simulink library "libMdl_GnssDataCorrector"  (R2019b)
settings: Solver=VariableStepAuto  StartTime=0.0  StopTime=10.0  RelTol=1e-3
undefined symbols (not defined in the file): gnss_lever_arm, sample_time
libraries: libMdl_transformVect x2, libMdl_crossProdMat x1
settings Model: Creator=Hanno  LastModifiedBy=Hanno

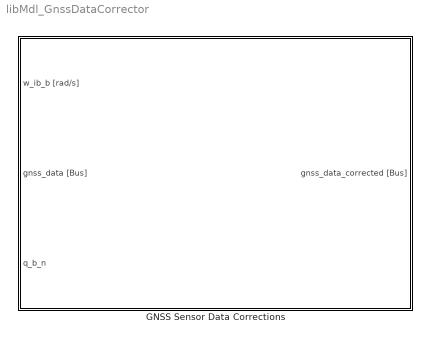
== system libMdl_GnssDataCorrector ==
  GNSS Sensor Data Corrections : Subsystem  mask(GNSS Sensor Data Corrections){mv_lever_arm=gnss_lever_arm, mv_sample_time=sample_time, mv_position_correction=on}
      mask prompts: mv_lever_arm "Lever Arm:"; mv_sample_time "Sample Time:"; mv_position_correction "Correct Position:"
      mask help: Lever Arm: Lever Arm Vector 'leverarm_s_b' in meters describing the mounting position of the sensor with respect to the body frame.
      mask Display:
      | if mv_position_correction
      |     pos_correction_str = 'on';
      | else
      |     pos_correction_str = 'off';
      | end % if
      | 
      | str1 = sprintf('\\color{black}{\\bfGNSS Data Correction}\n\n');
      | str2 = sprintf('Correct Position: %s\n',pos_correction_str);
      | str3 = sprintf('Sample Time: %0.3f',mv_sample_time);
      | 
      | str = [str1,str2,str3];
      | 
      | text( 0.5,0.5, ...
      |       str, ...
      |       'horizontalAlignment', 'center', ...
      |       'texmode','on' ...
      |     )

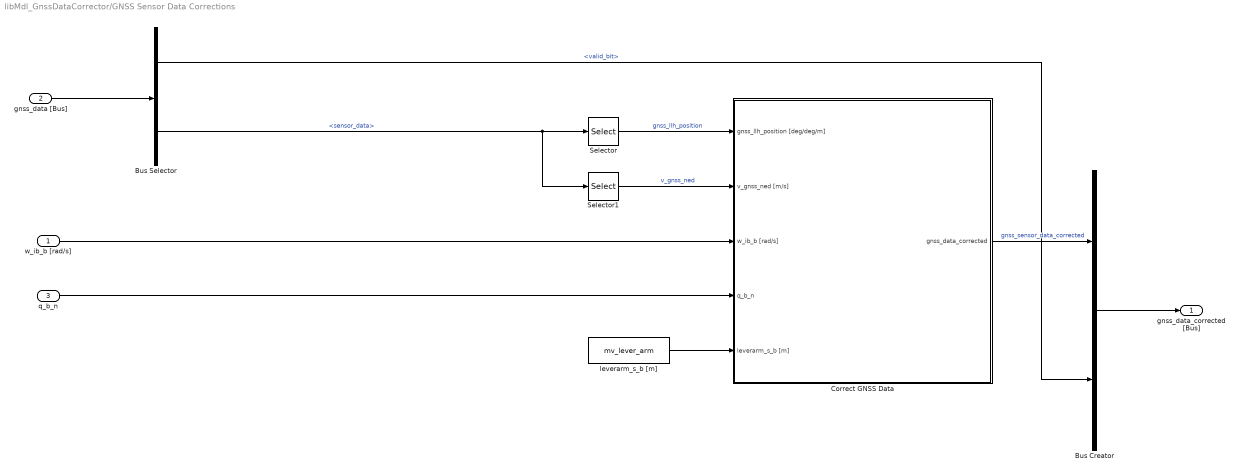
== system libMdl_GnssDataCorrector/GNSS Sensor Data Corrections ==
  w_ib_b [rad/s] : Inport
  gnss_data [Bus] : Inport  Port=2
  q_b_n : Inport  Port=3
  Bus Creator : BusCreator  Inputs=2
  Bus Selector : BusSelector  OutputSignals=valid_bit,sensor_data
  Correct GNSS Data : Subsystem  TreatAsAtomicUnit=on  SystemSampleTime=mv_sample_time
  Selector : Selector  InputPortWidth=7  IndexOptions=Index vector (dialog)  Indices=1:3  OutputSizes=1
  Selector1 : Selector  InputPortWidth=7  IndexOptions=Index vector (dialog)  Indices=4:6  OutputSizes=1
  leverarm_s_b [m] : Constant  Value=mv_lever_arm
  gnss_data_corrected [Bus] : Outport  VectorParamsAs1DForOutWhenUnconnected=off
  wires:
  gnss_data [Bus]/1 -> Bus Selector/1
  Bus Selector/2 -> Selector1/1, Selector/1  "<sensor_data>"
  Selector/1 -> Correct GNSS Data/1(gnss_llh_position [deg/deg/m])  "gnss_llh_position"
  Selector1/1 -> Correct GNSS Data/2(v_gnss_ned [m/s])  "v_gnss_ned"
  w_ib_b [rad/s]/1 -> Correct GNSS Data/3(w_ib_b [rad/s])
  q_b_n/1 -> Correct GNSS Data/4(q_b_n)
  leverarm_s_b [m]/1 -> Correct GNSS Data/5(leverarm_s_b [m])
  Bus Selector/1 -> Bus Creator/2  "<valid_bit>"
  Correct GNSS Data/1(gnss_data_corrected) -> Bus Creator/1  "gnss_sensor_data_corrected"
  Bus Creator/1 -> gnss_data_corrected [Bus]/1

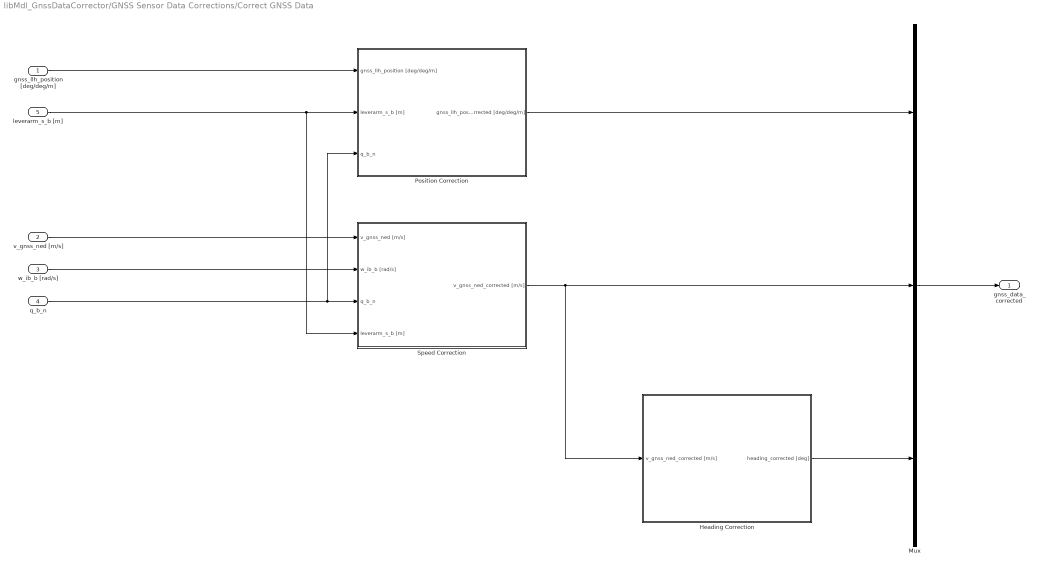
== system libMdl_GnssDataCorrector/GNSS Sensor Data Corrections/Correct GNSS Data ==
  gnss_llh_position [deg/deg/m] : Inport
  v_gnss_ned [m/s] : Inport  Port=2
  w_ib_b [rad/s] : Inport  Port=3
  q_b_n : Inport  Port=4
  leverarm_s_b [m] : Inport  Port=5
  Heading Correction : Subsystem
  Mux : Mux  Inputs=3
  Position Correction : Subsystem
  Speed Correction : Subsystem
  gnss_data_corrected : Outport
  wires:
  gnss_llh_position [deg/deg/m]/1 -> Position Correction/1(gnss_llh_position [deg/deg/m])
  Heading Correction/1(heading_corrected [deg]) -> Mux/3
  w_ib_b [rad/s]/1 -> Speed Correction/2(w_ib_b [rad/s])
  Speed Correction/1(v_gnss_ned_corrected [m/s]) -> Heading Correction/1(v_gnss_ned_corrected [m/s]), Mux/2
  Mux/1 -> gnss_data_corrected/1
  leverarm_s_b [m]/1 -> Position Correction/2(leverarm_s_b [m]), Speed Correction/4(leverarm_s_b [m])
  Position Correction/1(gnss_llh_position_corrected [deg/deg/m]) -> Mux/1
  q_b_n/1 -> Speed Correction/3(q_b_n), Position Correction/3(q_b_n)
  v_gnss_ned [m/s]/1 -> Speed Correction/1(v_gnss_ned [m/s])

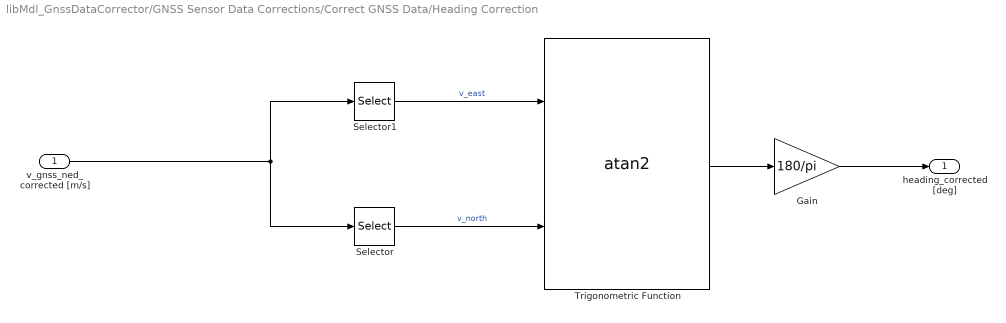
== system libMdl_GnssDataCorrector/GNSS Sensor Data Corrections/Correct GNSS Data/Heading Correction ==
  v_gnss_ned_corrected [m/s] : Inport
  Gain : Gain  Gain=180/pi
      settings: AttributesFormatString=rad2deg
  Selector : Selector  InputPortWidth=3  IndexOptions=Index vector (dialog)  Indices=1  OutputSizes=1
  Selector1 : Selector  InputPortWidth=3  IndexOptions=Index vector (dialog)  Indices=2  OutputSizes=1
  Trigonometric Function : Trigonometry  Operator=atan2
  heading_corrected [deg] : Outport
  wires:
  Trigonometric Function/1 -> Gain/1
  v_gnss_ned_corrected [m/s]/1 -> Selector1/1, Selector/1
  Selector1/1 -> Trigonometric Function/1  "v_east"
  Selector/1 -> Trigonometric Function/2  "v_north"
  Gain/1 -> heading_corrected [deg]/1

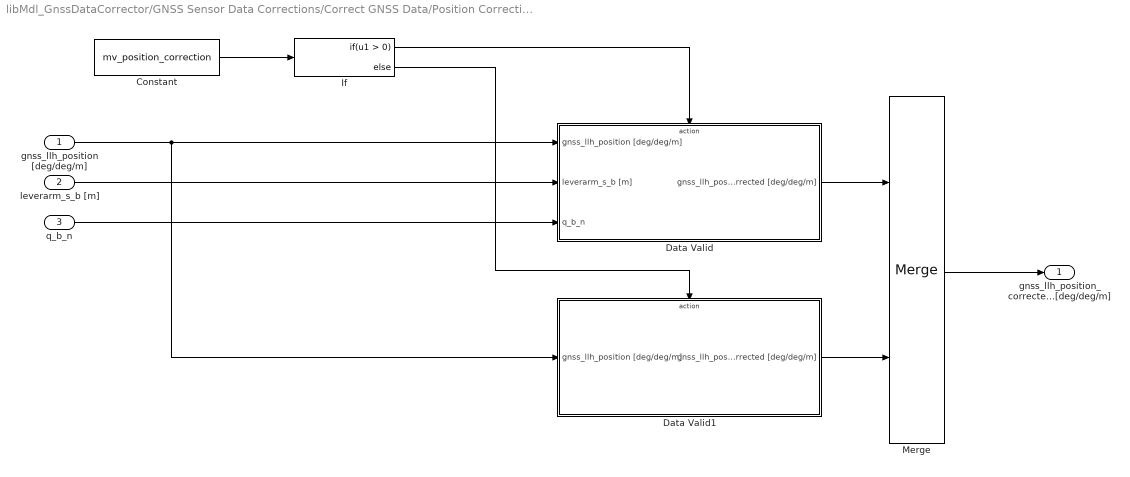
== system libMdl_GnssDataCorrector/GNSS Sensor Data Corrections/Correct GNSS Data/Position Correction ==
  gnss_llh_position [deg/deg/m] : Inport
  leverarm_s_b [m] : Inport  Port=2
  q_b_n : Inport  Port=3
  Constant : Constant  Value=mv_position_correction
  Data Valid : Subsystem  TreatAsAtomicUnit=on
  Data Valid1 : Subsystem  TreatAsAtomicUnit=on
  If : If
  Merge : Merge
  gnss_llh_position_corrected [deg/deg/m] : Outport
  wires:
  q_b_n/1 -> Data Valid/3(q_b_n)
  leverarm_s_b [m]/1 -> Data Valid/2(leverarm_s_b [m])
  gnss_llh_position [deg/deg/m]/1 -> Data Valid/1(gnss_llh_position [deg/deg/m]), Data Valid1/1(gnss_llh_position [deg/deg/m])
  If/2 -> Data Valid1/Action
  If/1 -> Data Valid/Action
  Constant/1 -> If/1
  Merge/1 -> gnss_llh_position_corrected [deg/deg/m]/1
  Data Valid1/1(gnss_llh_position_corrected [deg/deg/m]) -> Merge/2
  Data Valid/1(gnss_llh_position_corrected [deg/deg/m]) -> Merge/1

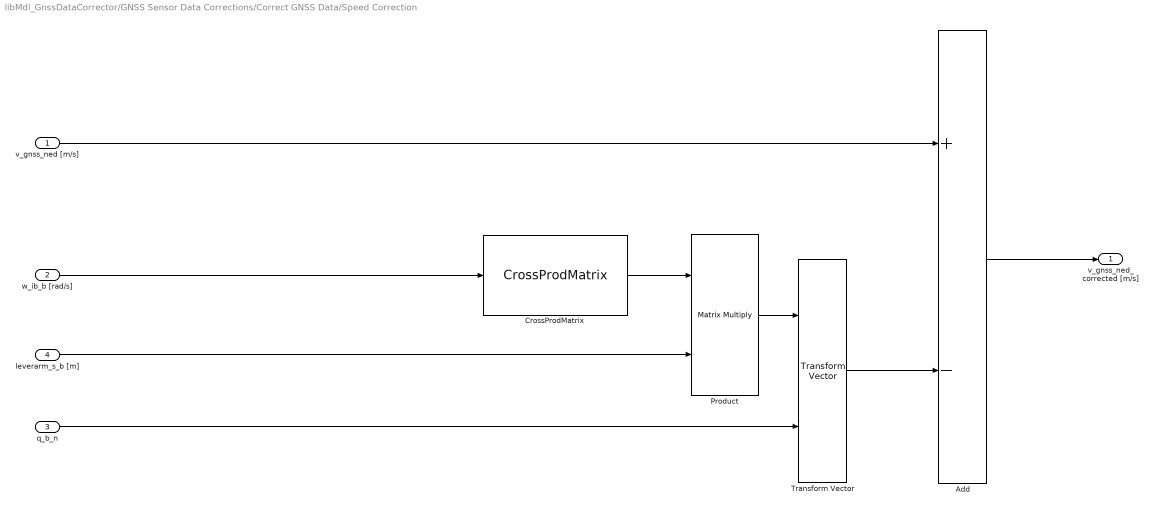
== system libMdl_GnssDataCorrector/GNSS Sensor Data Corrections/Correct GNSS Data/Speed Correction ==
  v_gnss_ned [m/s] : Inport
  w_ib_b [rad/s] : Inport  Port=2
  q_b_n : Inport  Port=3
  leverarm_s_b [m] : Inport  Port=4
  Add : Sum  Inputs=+-
  CrossProdMatrix : libMdl_crossProdMat/CrossProdMatrix  SystemSampleTime=-1  Latency=0  AutoFrameSizeCalculation=off
  Product : Product  Multiplication=Matrix(*)
  Transform Vector : libMdl_transformVect/Transform Vector  SystemSampleTime=-1  Latency=0  AutoFrameSizeCalculation=off
  v_gnss_ned_corrected [m/s] : Outport
  wires:
  Transform Vector/1 -> Add/2
  w_ib_b [rad/s]/1 -> CrossProdMatrix/1
  Add/1 -> v_gnss_ned_corrected [m/s]/1
  CrossProdMatrix/1 -> Product/1
  Product/1 -> Transform Vector/1
  q_b_n/1 -> Transform Vector/2
  v_gnss_ned [m/s]/1 -> Add/1
  leverarm_s_b [m]/1 -> Product/2

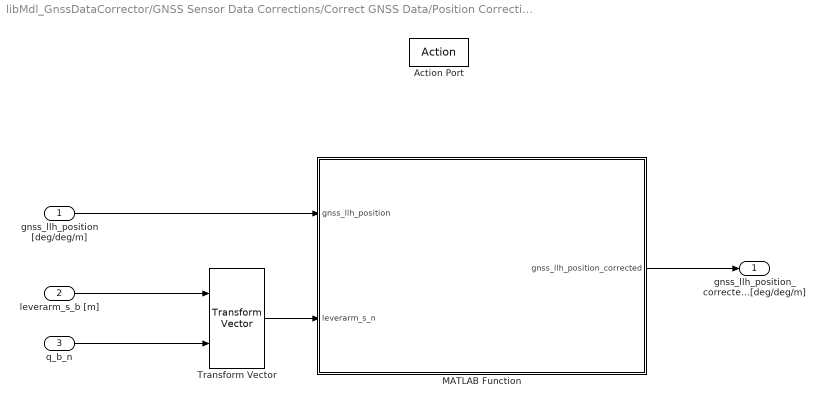
== system libMdl_GnssDataCorrector/GNSS Sensor Data Corrections/Correct GNSS Data/Position Correction/Data Valid ==
  gnss_llh_position [deg/deg/m] : Inport
  leverarm_s_b [m] : Inport  Port=2
  q_b_n : Inport  Port=3
  Action Port : ActionPort
  MATLAB Function : MATLAB Function  TreatAsAtomicUnit=on
  Transform Vector : libMdl_transformVect/Transform Vector  SystemSampleTime=-1  Latency=0  AutoFrameSizeCalculation=off
  gnss_llh_position_corrected [deg/deg/m] : Outport
  wires:
  q_b_n/1 -> Transform Vector/2
  gnss_llh_position [deg/deg/m]/1 -> MATLAB Function/1(gnss_llh_position)
  Transform Vector/1 -> MATLAB Function/2(leverarm_s_n)
  MATLAB Function/1(gnss_llh_position_corrected) -> gnss_llh_position_corrected [deg/deg/m]/1
  leverarm_s_b [m]/1 -> Transform Vector/1

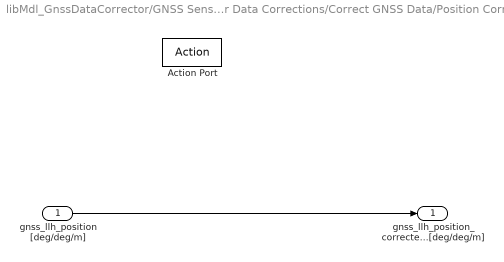
== system libMdl_GnssDataCorrector/GNSS Sensor Data Corrections/Correct GNSS Data/Position Correction/Data Valid1 ==
  gnss_llh_position [deg/deg/m] : Inport
  Action Port : ActionPort
  gnss_llh_position_corrected [deg/deg/m] : Outport
  wires:
  gnss_llh_position [deg/deg/m]/1 -> gnss_llh_position_corrected [deg/deg/m]/1

== matlab function libMdl_GnssDataCorrector/GNSS Sensor Data Corrections/Correct GNSS Data/Position Correction/Data Valid/MATLAB Function ==
  data: gnss_llh_position input; leverarm_s_n input; gnss_llh_position_corrected output
function gnss_llh_position_corrected = gnssOffsetCorrection(gnss_llh_position,leverarm_s_n)

gnss_llh_position_corrected = coder.nullcopy(zeros(3,1));

persistent mem_var_utm_zone
 
%% Calculations

if isempty(mem_var_utm_zone)
    [x,y,f] = ll2utm_stripped(gnss_llh_position(1),gnss_llh_position(2));
    mem_var_utm_zone = f;
else
    [x,y] = ll2utm_stripped(gnss_llh_position(1),gnss_llh_position(2),mem_var_utm_zone);
    f = mem_var_utm_zone;
end % if
p_gnss_utm = [x;y;gnss_llh_position(3)];

p_corrected_utm = p_gnss_utm - [0 1 0;1 0 0;0 0 -1]*leverarm_s_n(:);

x_corrected = p_corrected_utm(1);
y_corrected = p_corrected_utm(2);
z_corrected = p_corrected_utm(3);

[lat,lon] = utm2ll_stripped(x_corrected,y_corrected,f);

gnss_llh_position_corrected = [lat;lon;z_corrected];

end % if
